simulink model "ControllersComparison"  (R2019b)
settings: Solver=VariableStepAuto  StartTime=0.0  StopTime=tsim  MaxStep=0.01  RelTol=1e-3
values from neighbouring files (symbols this model uses):
  IC = [64.828,     0,  -0.0153, 0,  0,  0,     0, 0,   0,     0,    0, 1119]    [AF_Sim_Init.m]
libraries: simulink_extras x10, simulink x2, aerolibanim x1
settings Model: Creator=Victor  LastModifiedBy=Victor
settings SolverCC: MaxConsecutiveMinStep=50

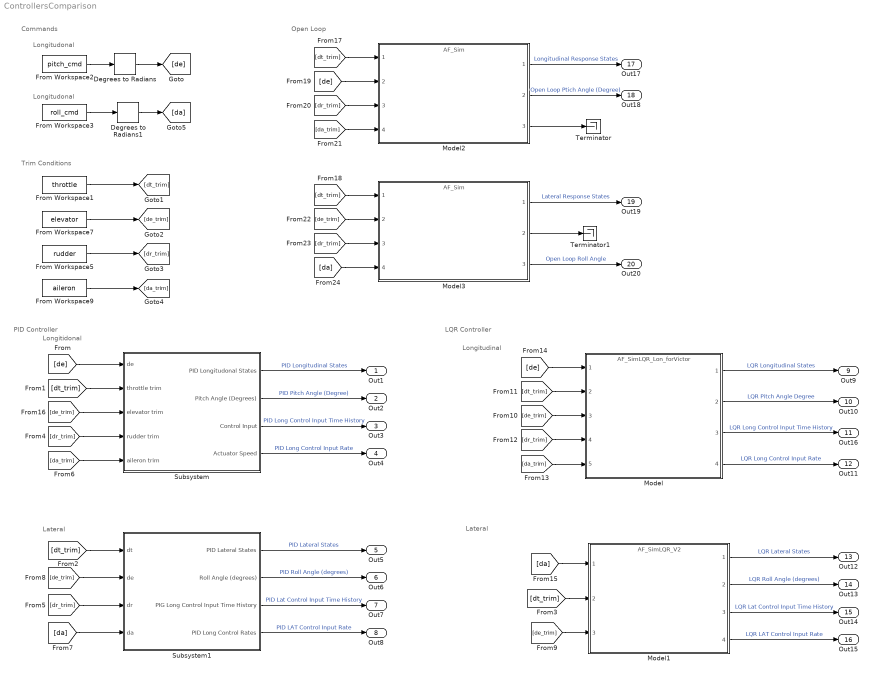
== system ControllersComparison ==
  note: Open Loop
  note: Trim Conditions
  note: Longitudonal
  note: Commands
  note: Longitidonal
  note: PID Controller
  note: Lateral
  note: Longitudinal
  note: LQR Controller
  note: Lateral
  note: Longitudonal
  Degrees to Radians : simulink_extras/Transformations/Degrees to Radians
  Degrees to Radians1 : simulink_extras/Transformations/Degrees to Radians
  From Workspace1 : FromWorkspace  VariableName=throttle  SampleTime=0
  From Workspace2 : FromWorkspace  VariableName=pitch_cmd  SampleTime=0
  From Workspace3 : FromWorkspace  VariableName=roll_cmd  SampleTime=0
  From Workspace5 : FromWorkspace  VariableName=rudder  SampleTime=0
  From Workspace7 : FromWorkspace  VariableName=elevator  SampleTime=0
  From Workspace9 : FromWorkspace  VariableName=aileron  SampleTime=0
  Model : ModelReference  ModelNameDialog=AF_SimLQR_Lon_forVictor.slx  SimulationMode=Normal  ModelReferenceVersion=1.103
  Model1 : ModelReference  ModelNameDialog=AF_SimLQR_V2.slx  SimulationMode=Normal  ModelReferenceVersion=1.56
  Model2 : ModelReference  ModelNameDialog=AF_Sim.slx  SimulationMode=Normal  ModelReferenceVersion=1.35
  Model3 : ModelReference  ModelNameDialog=AF_Sim.slx  SimulationMode=Normal  ModelReferenceVersion=1.35
  Subsystem : Subsystem
  Subsystem1 : Subsystem
  Terminator : Terminator
  Terminator1 : Terminator
  Out1 : Outport
  Out2 : Outport  Port=2
  Out3 : Outport  Port=3
  Out4 : Outport  Port=4
  Out5 : Outport  Port=5
  Out6 : Outport  Port=6
  Out7 : Outport  Port=7
  Out8 : Outport  Port=8
  Out9 : Outport  Port=9
  Out10 : Outport  Port=10
  Out16 : Outport  Port=11
  Out11 : Outport  Port=12
  Out12 : Outport  Port=13
  Out13 : Outport  Port=14
  Out14 : Outport  Port=15
  Out15 : Outport  Port=16
  Out17 : Outport  Port=17
  Out18 : Outport  Port=18
  Out19 : Outport  Port=19
  Out20 : Outport  Port=20
  wires:
  Subsystem/1(PID Longitudonal States) -> Out1/1  "PID Longitudinal States"
  Subsystem/2(Pitch Angle (Degrees)) -> Out2/1  "PID Pitch Angle (Degree)"
  Subsystem/3(Control Input) -> Out3/1  "PID Long Control Input Time History"
  Subsystem/4(Actuator Speed) -> Out4/1  "PID Long Control Input Rate"
  Subsystem1/1(PID Lateral States) -> Out5/1  "PID Lateral States"
  Subsystem1/2(Roll Angle (degrees)) -> Out6/1  "PID Roll Angle (degrees)"
  Subsystem1/3(PIG Long Control Input Time History) -> Out7/1  "PID Lat Control Input Time History"
  Subsystem1/4(PID Long Control Rates) -> Out8/1  "PID LAT Control Input Rate"
  From Workspace2/1 -> Degrees to Radians/1
  Degrees to Radians/1 -> [de]
  [de] -> Subsystem/1(de)
  From Workspace1/1 -> [dt_trim]
  From Workspace7/1 -> [de_trim]
  From Workspace5/1 -> [dr_trim]
  From Workspace9/1 -> [da_trim]
  [dt_trim] -> Subsystem/2(throttle trim)
  [dt_trim] -> Subsystem1/1(dt)
  [dr_trim] -> Subsystem/4(rudder trim)
  [dr_trim] -> Subsystem1/3(dr)
  [da_trim] -> Subsystem/5(aileron trim)
  From Workspace3/1 -> Degrees to Radians1/1
  Degrees to Radians1/1 -> [da]
  [da] -> Subsystem1/4(da)
  [de_trim] -> Subsystem1/2(de)
  [dt_trim] -> Model/2
  [dr_trim] -> Model/4
  [da_trim] -> Model/5
  [de] -> Model/1
  Model/1 -> Out9/1  "LQR Longitudinal States"
  Model/2 -> Out10/1  "LQR Pitch Angle Degree"
  Model/3 -> Out16/1  "LQR Long Control Input Time History"
  Model/4 -> Out11/1  "LQR Long Control Input Rate"
  [de_trim] -> Model/3
  Model1/4 -> Out15/1  "LQR LAT Control Input Rate"
  Model1/3 -> Out14/1  "LQR Lat Control Input Time History"
  Model1/2 -> Out13/1  "LQR Roll Angle (degrees)"
  Model1/1 -> Out12/1  "LQR Lateral States"
  [da] -> Model1/1
  [dt_trim] -> Model1/2
  [de_trim] -> Model1/3
  [de_trim] -> Subsystem/3(elevator trim)
  [dt_trim] -> Model2/1
  [dt_trim] -> Model3/1
  [de] -> Model2/2
  [dr_trim] -> Model2/3
  [da_trim] -> Model2/4
  [de_trim] -> Model3/2
  [dr_trim] -> Model3/3
  [da] -> Model3/4
  Model2/1 -> Out17/1  "Longitudinal Response States"
  Model2/2 -> Out18/1  "Open Loop Ptich Angle (Degree)"
  Model2/3 -> Terminator/1
  Model3/1 -> Out19/1  "Lateral Response States"
  Model3/2 -> Terminator1/1
  Model3/3 -> Out20/1  "Open Loop Roll Angle"

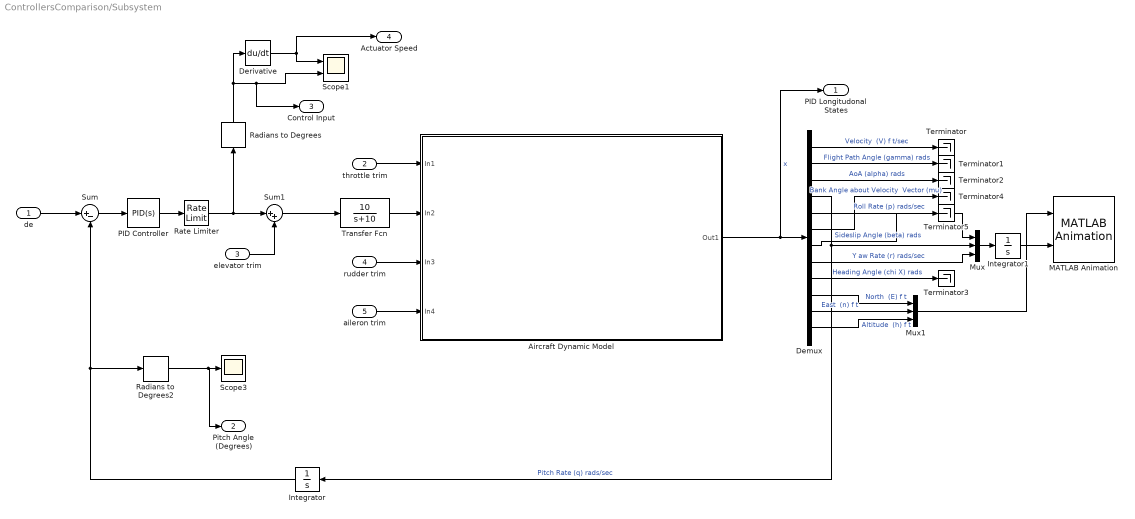
== system ControllersComparison/Subsystem ==
  de : Inport
  throttle trim : Inport  Port=2
  elevator trim : Inport  Port=3
  rudder trim : Inport  Port=4
  aileron trim : Inport  Port=5
  Aircraft Dynamic Model : Subsystem
  Demux : Demux  Outputs=12
  Derivative : Derivative
  Integrator : Integrator
  Integrator1 : Integrator
  MATLAB Animation : aerolibanim/MATLAB Animation  Tag=Matlab Animation 6 DOF  Vehicles=1  Geometries='astredwedge.mat'  BoundingBoxCoordinates=[-50,50,-50,50,-50,50]  CameraOffset=[100,100,100]  CameraViewAngle=4  SampleTime=0.2  FigurePosition=[403,303,275,214]
      settings: SourceProductName=Aerospace Blockset  SourceProductBaseCode=AE
  Mux : Mux  Inputs=3
  Mux1 : Mux  Inputs=3
  PID Controller : simulink/Continuous/PID Controller  Controller=PID  Form=Parallel  TimeDomain=Continuous-time  SampleTime=-1  IntegratorMethod=Forward Euler  FilterMethod=Forward Euler  ControllerParametersSource=internal  P=-1.49308929498648  I=-1.41849985038044  D=-0.103757248214564  UseFilter=on  N=316.418420565516  TunerSelectOption=Transfer Function Based (PID Tuner App)  InitialConditionSource=internal  InitialConditionForIntegrator=0  InitialConditionForFilter=0  DifferentiatorICPrevScaledInput=0  ExternalReset=none  TrackingMode=off  Kt=1  LimitOutput=off  UpperSaturationLimit=12*(pi/180)  LowerSaturationLimit=-12*(pi/180)  LinearizeAsGain=off  AntiWindupMode=back-calculation  Kb=-3  POutMin=[]  POutMax=[]  IOutMin=[]  IOutMax=[]  DOutMin=[]  DOutMax=[]  NOutMin=[]  NOutMax=[]  SumOutMin=[]  SumOutMax=[]  SaturationOutMin=[]  SaturationOutMax=[]  PParamMin=[]  PParamMax=[]  IParamMin=[]  IParamMax=[]  DParamMin=[]  DParamMax=[]  NParamMin=[]  NParamMax=[]  KbParamMin=[]  KbParamMax=[]  KtParamMin=[]  KtParamMax=[]  KbOutMin=[]  KbOutMax=[]  KtOutMin=[]  KtOutMax=[]  IntegratorOutMin=[]  IntegratorOutMax=[]  FilterOutMin=[]  FilterOutMax=[]  SumI1OutMin=[]  SumI1OutMax=[]  SumI2OutMin=[]  SumI2OutMax=[]  SumI3OutMin=[]  SumI3OutMax=[]  SumI4OutMin=[]  SumI4OutMax=[]  SumDOutMin=[]  SumDOutMax=[]  DifferentiatorOutMin=[]  DifferentiatorOutMax=[]  FilterDiffOutCoefMin=[]  FilterDiffOutCoefMax=[]  ReciprocalOutMin=[]  ReciprocalOutMax=[]  SumDenOutMin=[]  SumDenOutMax=[]  SumNumOutMin=[]  SumNumOutMax=[]  DivideOutMin=[]  DivideOutMax=[]  IntegratorContinuousStateAttributes=''  IntegratorStateMustResolveToSignalObject=off  IntegratorRTWStateStorageClass=Auto  FilterContinuousStateAttributes=''  FilterStateMustResolveToSignalObject=off  FilterRTWStateStorageClass=Auto  ParallelPVariant=InternalParameters  IdealPVariant=Disabled  IVariant=InternalParameters  DVariant=InternalParameters  IntegratorVariant=Continuous  SatVariant=Disabled  AWVariant=Passthrough  PCopyVariant=Disabled  TRVariant=Disabled  FdbkBlocksVariant=Forward  IdealPFdbkVariant=Disabled  SatFdbkVariant=Disabled  DerivativeFilterVariant=ContFilter  NVariant=InternalParameters  NCopyVariant=Disabled  FilterICVariant=InternalICsFilter  IntegratorICVariant=InternalICs  ExternalResetVariant=Disabled  TRSumVariant=Passthrough  SumFdbkVariant=Disabled  SumVariant=Sum_PID
  Radians to Degrees : simulink_extras/Transformations/Radians to Degrees
  Radians to Degrees2 : simulink_extras/Transformations/Radians to Degrees
  Rate Limiter : RateLimiter  RisingSlewLimit=10  FallingSlewLimit=-10  SampleTimeMode=inherited
  Scope1 : Scope  NumInputPorts=2
  Scope3 : Scope
  Sum : Sum  Inputs=|+-
  Sum1 : Sum  Inputs=|++
  Terminator{,1..5} (6 alike) : Terminator
  Transfer Fcn : TransferFcn  Numerator=[10]  Denominator=[1 10]
  PID Longitudonal States : Outport
  Pitch Angle (Degrees) : Outport  Port=2
  Control Input : Outport  Port=3
  Actuator Speed : Outport  Port=4
  wires:
  Aircraft Dynamic Model/1(Out1) -> PID Longitudonal States/1, Demux/1  "x"
  Demux/4 -> Integrator/1, Mux/2  "Pitch Rate (q) rads/sec"
  Sum/1 -> PID Controller/1
  Transfer Fcn/1 -> Aircraft Dynamic Model/2(In2)
  Derivative/1 -> Scope1/1, Actuator Speed/1
  Radians to Degrees/1 -> Derivative/1, Control Input/1, Scope1/2
  rudder trim/1 -> Aircraft Dynamic Model/3(In3)
  aileron trim/1 -> Aircraft Dynamic Model/4(In4)
  throttle trim/1 -> Aircraft Dynamic Model/1(In1)
  de/1 -> Sum/1
  Integrator/1 -> Sum/2, Radians to Degrees2/1
  Radians to Degrees2/1 -> Pitch Angle (Degrees)/1, Scope3/1
  Demux/5 -> Mux/1  "Roll Rate (p) rads/sec"
  Demux/8 -> Mux/3  "Y aw Rate (r) rads/sec"
  Mux/1 -> Integrator1/1
  Integrator1/1 -> MATLAB Animation/2
  Demux/10 -> Mux1/1  "North  (E) f t"
  Demux/11 -> Mux1/2  "East  (n) f t"
  Demux/12 -> Mux1/3  "Altitude  (h) f t"
  Mux1/1 -> MATLAB Animation/1
  Sum1/1 -> Transfer Fcn/1
  Demux/1 -> Terminator/1  "Velocity  (V) f t/sec"
  Demux/2 -> Terminator1/1  "Flight Path Angle (gamma) rads"
  Demux/3 -> Terminator2/1  "AoA (alpha) rads"
  Demux/9 -> Terminator3/1  "Heading Angle (chi X) rads"
  Demux/6 -> Terminator4/1  "Bank Angle about Velocity  Vector (mu)"
  Demux/7 -> Terminator5/1  "Sideslip Angle (beta) rads"
  elevator trim/1 -> Sum1/2
  Rate Limiter/1 -> Radians to Degrees/1, Sum1/1
  PID Controller/1 -> Rate Limiter/1

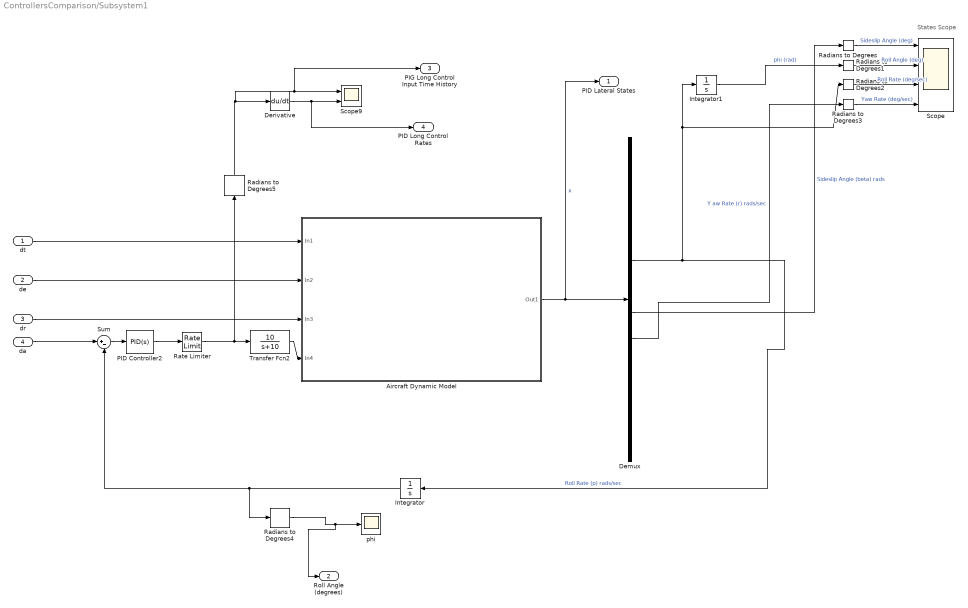
== system ControllersComparison/Subsystem1 ==
  note: States Scope
  dt : Inport
  de : Inport  Port=2
  dr : Inport  Port=3
  da : Inport  Port=4
  Aircraft Dynamic Model : Subsystem
  Demux : Demux  Outputs=12
  Derivative : Derivative
  Integrator : Integrator
  Integrator1 : Integrator
  PID Controller2 : simulink/Continuous/PID Controller  Controller=PID  Form=Parallel  TimeDomain=Continuous-time  SampleTime=-1  IntegratorMethod=Forward Euler  FilterMethod=Forward Euler  ControllerParametersSource=internal  P=1.61606482849741  I=1.22173294294368  D=0.356576763881949  UseFilter=on  N=1149.82034893271  TunerSelectOption=Transfer Function Based (PID Tuner App)  InitialConditionSource=internal  InitialConditionForIntegrator=0  InitialConditionForFilter=0  DifferentiatorICPrevScaledInput=0  ExternalReset=none  TrackingMode=off  Kt=1  LimitOutput=off  UpperSaturationLimit=inf  LowerSaturationLimit=-inf  LinearizeAsGain=on  AntiWindupMode=none  Kb=1  POutMin=[]  POutMax=[]  IOutMin=[]  IOutMax=[]  DOutMin=[]  DOutMax=[]  NOutMin=[]  NOutMax=[]  SumOutMin=[]  SumOutMax=[]  SaturationOutMin=[]  SaturationOutMax=[]  PParamMin=[]  PParamMax=[]  IParamMin=[]  IParamMax=[]  DParamMin=[]  DParamMax=[]  NParamMin=[]  NParamMax=[]  KbParamMin=[]  KbParamMax=[]  KtParamMin=[]  KtParamMax=[]  KbOutMin=[]  KbOutMax=[]  KtOutMin=[]  KtOutMax=[]  IntegratorOutMin=[]  IntegratorOutMax=[]  FilterOutMin=[]  FilterOutMax=[]  SumI1OutMin=[]  SumI1OutMax=[]  SumI2OutMin=[]  SumI2OutMax=[]  SumI3OutMin=[]  SumI3OutMax=[]  SumI4OutMin=[]  SumI4OutMax=[]  SumDOutMin=[]  SumDOutMax=[]  DifferentiatorOutMin=[]  DifferentiatorOutMax=[]  FilterDiffOutCoefMin=[]  FilterDiffOutCoefMax=[]  ReciprocalOutMin=[]  ReciprocalOutMax=[]  SumDenOutMin=[]  SumDenOutMax=[]  SumNumOutMin=[]  SumNumOutMax=[]  DivideOutMin=[]  DivideOutMax=[]  IntegratorContinuousStateAttributes=''  IntegratorStateMustResolveToSignalObject=off  IntegratorRTWStateStorageClass=Auto  FilterContinuousStateAttributes=''  FilterStateMustResolveToSignalObject=off  FilterRTWStateStorageClass=Auto  ParallelPVariant=InternalParameters  IdealPVariant=Disabled  IVariant=InternalParameters  DVariant=InternalParameters  IntegratorVariant=Continuous  SatVariant=Disabled  AWVariant=Passthrough  PCopyVariant=Disabled  TRVariant=Disabled  FdbkBlocksVariant=Forward  IdealPFdbkVariant=Disabled  SatFdbkVariant=Disabled  DerivativeFilterVariant=ContFilter  NVariant=InternalParameters  NCopyVariant=Disabled  FilterICVariant=InternalICsFilter  IntegratorICVariant=InternalICs  ExternalResetVariant=Disabled  TRSumVariant=Passthrough  SumFdbkVariant=Disabled  SumVariant=Sum_PID
  Radians to Degrees{,1..5} (6 alike) : simulink_extras/Transformations/Radians to Degrees
  Rate Limiter : RateLimiter  RisingSlewLimit=10  FallingSlewLimit=-10  SampleTimeMode=inherited
  Scope : Scope  NumInputPorts=4
  Scope9 : Scope  NumInputPorts=2
  Sum : Sum  Inputs=|+-
  Transfer Fcn2 : TransferFcn  Numerator=[10]  Denominator=[1 10]
  phi : Scope
  PID Lateral States : Outport
  Roll Angle (degrees) : Outport  Port=2
  PIG Long Control Input Time History : Outport  Port=3
  PID Long Control Rates : Outport  Port=4
  wires:
  Demux/8 -> Radians to Degrees3/1  "Y aw Rate (r) rads/sec"
  Aircraft Dynamic Model/1(Out1) -> PID Lateral States/1, Demux/1  "x"
  Rate Limiter/1 -> Transfer Fcn2/1, Radians to Degrees5/1
  Derivative/1 -> PID Long Control Rates/1, Scope9/2
  Demux/5 -> Radians to Degrees2/1, Integrator1/1, Integrator/1  "Roll Rate (p) rads/sec"
  dt/1 -> Aircraft Dynamic Model/1(In1)
  Demux/7 -> Radians to Degrees/1  "Sideslip Angle (beta) rads"
  Radians to Degrees4/1 -> Roll Angle (degrees)/1, phi/1
  Integrator1/1 -> Radians to Degrees1/1  "phi (rad)"
  dr/1 -> Aircraft Dynamic Model/3(In3)
  Radians to Degrees3/1 -> Scope/4  "Yaw Rate (deg/sec)"
  Radians to Degrees1/1 -> Scope/2  "Roll Angle (deg)"
  Radians to Degrees/1 -> Scope/1  "Sideslip Angle (deg)"
  Transfer Fcn2/1 -> Aircraft Dynamic Model/4(In4)
  de/1 -> Aircraft Dynamic Model/2(In2)
  Radians to Degrees2/1 -> Scope/3  "Roll Rate (deg/sec)"
  Sum/1 -> PID Controller2/1
  PID Controller2/1 -> Rate Limiter/1
  Integrator/1 -> Radians to Degrees4/1, Sum/2
  da/1 -> Sum/1
  Radians to Degrees5/1 -> Derivative/1, PIG Long Control Input Time History/1, Scope9/1

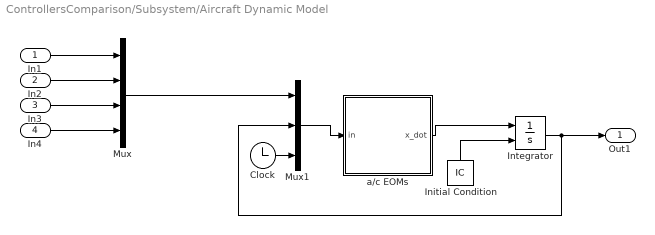
== system ControllersComparison/Subsystem/Aircraft Dynamic Model ==
  In1 : Inport
  In2 : Inport  Port=2
  In3 : Inport  Port=3
  In4 : Inport  Port=4
  Clock : Clock
      settings: Decimation=100
  Initial Condition : Constant  Value=IC
  Integrator : Integrator  InitialConditionSource=external
  Mux : Mux
  Mux1 : Mux  Inputs=3
  a/c EOMs : MATLAB Function  TreatAsAtomicUnit=on
  Out1 : Outport  VectorParamsAs1DForOutWhenUnconnected=off
  wires:
  Initial Condition/1 -> Integrator/2
  Clock/1 -> Mux1/3
  Integrator/1 -> Mux1/2, Out1/1
  Mux1/1 -> a/c EOMs/1(in)
  a/c EOMs/1(x_dot) -> Integrator/1
  Mux/1 -> Mux1/1
  In1/1 -> Mux/1
  In2/1 -> Mux/2
  In3/1 -> Mux/3
  In4/1 -> Mux/4

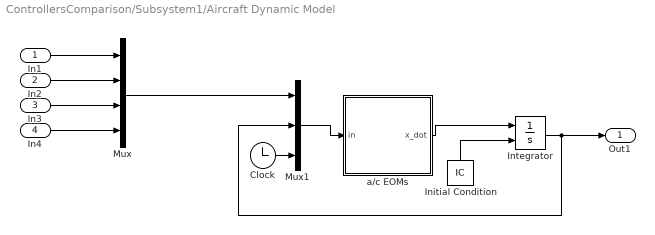
== system ControllersComparison/Subsystem1/Aircraft Dynamic Model ==
  In1 : Inport
  In2 : Inport  Port=2
  In3 : Inport  Port=3
  In4 : Inport  Port=4
  Clock : Clock
      settings: Decimation=100
  Initial Condition : Constant  Value=IC
  Integrator : Integrator  InitialConditionSource=external
  Mux : Mux
  Mux1 : Mux  Inputs=3
  a/c EOMs : MATLAB Function  TreatAsAtomicUnit=on
  Out1 : Outport  VectorParamsAs1DForOutWhenUnconnected=off
  wires:
  a/c EOMs/1(x_dot) -> Integrator/1
  In3/1 -> Mux/3
  Clock/1 -> Mux1/3
  Integrator/1 -> Mux1/2, Out1/1
  Initial Condition/1 -> Integrator/2
  Mux/1 -> Mux1/1
  Mux1/1 -> a/c EOMs/1(in)
  In4/1 -> Mux/4
  In2/1 -> Mux/2
  In1/1 -> Mux/1

== matlab function ControllersComparison/Subsystem1/Aircraft Dynamic Model/a//c EOMs ==
  data: in input; x_dot output
function x_dot  = fcn(in)

%global manuever alpha_dot;
x_dot = zeros(12,1);

alpha_dot = 0;

%temporary input vector
%u0 = [1.29, -0.1174, 0,  0, 64.828,     0,  -0.0153, 0,  0,  0,     0, 0,   0,     0,    0, 1119, 100];
    % [T,     de,    dr, da, V,      gamma,  AoA,     q,  p, mu,  beta, r, chi, north, east,    h, clock-input]
  
%in = u0;

% PARSING INPUTS
%=============================================================
T   = in(1); %Thrust
de  = in(2); %Elevator deflection (down is +) {deg}
drt = in(3); %Rudder deflection {deg}
da  = in(4); %Aileron deflection {deg}

V       = in(5);  %Velocity {ft/s}
gamma   = in(6);  %Flight path angle {rad}
alpha   = in(7);  %Angle of attack {rad}
q       = in(8);  %Pitch Rate {rad/s}
p       = in(9);  %Roll Rate {rad/s}
mu      = in(10); %Bank Angle (About Velocity Vector) {rad}
beta    = in(11); %Sideslip Angle {rad}
r       = in(12); %Yaw Rate {rad/s}
chi     = in(13); %Heading angle {rads}
north   = in(14); %North Position {ft}
east    = in(15); %East Position {ft}
h       = in(16); %Altitude {ft}
tm = in(17); % time {s}

% ATMOSPHERIC PROPERTIES
%=============================================================
rho = 0.0023081;    %Air Density (slugs per ft^3) -> do we want to make this a function of height?
g = 32.17;          %ft/s^2


% AIRCRAFT PROPERTIES
%==============================================================


m = 0.487669;       %Slugs - empty mass w/o fuel
Iyy = 1.5523;       %Inertia found with empty mass
Ixx = 1.948;        %Inertia
Izz = 1.9166;       %Inertia
Ixz = 0;            %Assumed zero due to symmetric aircraft

S = 10.56;          %Wing area - square feet
b = 9.16;           % Wing span - feet

CLow = 0.421;       %Wing coefficient of lift at 0deg AoA
CLaw = 4.59;        %Wing coefficient of lift per AoA
CDminw = 0.011;     %wing minimum coefficient of drag
ARw = (b^2)/S;      %Wing aspect ratio
e = 0.75;           %Span efficiency - ESTIMATION
Kw = 1/(pi*ARw*e);  %
Cmw = -0.005;       %Wing moment coefficient
cgw = -(5/12);      %Distance aero center is back from cg - 5 inches
c = (16/12);        %Root chord of wing (16") - feet
lambda = 0.72955;   %Taper ratio from S = (Cr*(1+lambda)*b)/2
CLat = 0.76;        %Vert tail coefficient of lift per AoA
CDmint = 0.002;     %vert tail minimum coeffcient of drag
Kt = 0.446;         %TO DO - MORE CALC?
it = deg2rad(2);    %Tail incidence 2 degrees to radians
Te = 0.422;         %Tail control surface effectiveness (??)
nt = 1;             %??
St = S;             %Horizontal tail area square feet = ref area (??)
cgt = 3.5;          %Distance tail aero center back from a/c cg

CLavt = 0.0969;     %Vertical tail coefficient of lift per AoA(??)
CDminvt = 0.001;    %vert tail min coefficient of drag (??)
Svt = S;            %Ref area of vertical tail = ref area (??)
Tr = 0.434;         %Name??
nvt = nt;           %same as hori tail (??)
cgvt = cgt;         %same as hori tail (??)

Cmaf = 0.114;       %fuselage moment coefficient
CDf = 0.005;        %Fuselage coefficient of drag

Cnda = -0.0128;     %per rad (??)
Clda = 0.244;       %per rad (??)

%Eqns 17-25
CLw=CLow+CLaw*alpha;
CDw=CDminw+Kw*CLw^2;
E=2*(CLow+CLaw*(alpha-alpha_dot*(cgt+cgw)/V))/(pi*ARw);
alphat=alpha+it+Te*de+q*cgt/V-E;
CLt=CLat*alphat;
CDt=CDmint+Kt*CLt^2;
Cmf=Cmaf*alpha;
CDvt=CDminvt;
Clp=-1/12*CLaw*(1+3*lambda)/(1+lambda);

Clb=-.1;
Clr=.01;

%Eqns 26 - 33
qb=.5*rho*V^2;
Lw=qb*S*CLw;
Dw=qb*S*CDw;
Mw=qb*S*c*Cmw;
Lt=nt*qb*St*CLt;
Dt=nt*qb*St*CDt;
Df=qb*S*CDf;
Mf=qb*S*c*Cmf;
Dvt=nt*qb*Svt*CDvt;

% Calculate Forces and Moments
% Lift
L=Lw+Lt*cos(E-q*cgt/V)-(Dt+Dvt)*sin(E-q*cgt/V);
% Drag
D=Dw+(Dt+Dvt)*cos(E-q*cgt/V)+Lt*sin(E-q*cgt/V)+Df;
% Side Force
Y=nvt*qb*Svt*CLavt*(-beta+Tr*drt+r*cgvt/V);
% Pitch Moment
Mc=Lw*cgw*cos(alpha)+Dw*cgw*sin(alpha)+Mw-Lt*cgt*cos(alpha-E+q*cgt/V)-(Dt+Dvt)*cgt*sin(alpha-E+q*cgt/V)+Mf;
% Yaw Moment
Nc=-qb*nvt*Svt*CLavt*(-beta+Tr*drt+r*cgvt/V)*cgvt+(-qb*S*b*Cnda*da);
% Roll Moment
Lc=qb*S*b^2/(2*V)*(Clp*p+2*V/b*Clb*beta+Clr*drt+Clda*da*2*V/b);

% -=-=-=-=-=- NONLINEAR 6-DOF EQUATION OF MOTION (EOMs) -=-=-=-=-=-=-=-=-
%
% These are the state derivative equations; the comment names the state,
% but the equation is for its derivative (rate)
%
% The equations are arranged by aircraft mode
%
% NOTE: These assume that Ixz=0, if not, then eq's need to be modified
% Longitudinal (phugoid and short period): V, gamma, q, alpha
% Phugoid: V, gamma
 % Velocity
 V_dot=1/m*(-D*cos(beta)+Y*sin(beta)+T*cos(beta)*cos(alpha))-...
 g*sin(gamma);
 % Flight Path Angle
 gamma_dot=1/(m*V)*(-D*sin(beta)*sin(mu)-Y*sin(mu)*cos(beta)...
 +L*cos(mu)+T*(cos(mu)*sin(alpha)+sin(mu)*sin(beta)*cos(alpha)))...
 -g/V*cos(gamma);
% Short Period: alpha, q
 % Angle of Attach
 alpha_dot=q-tan(beta)*(p*cos(alpha)+r*sin(alpha))-1/(m*V*cos(beta))...
 *(L+T*sin(alpha))+g*cos(gamma)*cos(mu)/(V*cos(beta));
 % Pitch Rate
 q_dot=Mc/Iyy+1/Iyy*(Izz*p*r-Ixx*r*p);
% Lateral (roll) - Directional (yaw): p, mu, beta, r
% Roll: p, mu
 % Roll Rate
 p_dot=Lc/Ixx+1/Ixx*(Iyy*r*q-Izz*q*r);

 % Bank Angle (about velocity vector)
 mu_dot=1/cos(beta)*(p*cos(alpha)+r*sin(alpha))+1/(m*V)*(D*sin(beta)...
 *cos(mu)*tan(gamma)+Y*tan(gamma)*cos(mu)*cos(beta)+L*(tan(beta)+...
 tan(gamma)*sin(mu))+T*(sin(alpha)*tan(gamma)*sin(mu)+sin(alpha)*...
 tan(beta)-cos(alpha)*tan(gamma)*cos(mu)*sin(beta)))-...
 g/V*cos(gamma)*cos(mu)*tan(beta);

% Dutch Roll: beta, r
 % Side Slip Angle
 beta_dot=-r*cos(alpha)+p*sin(alpha)+1/(m*V)*(D*sin(beta)+Y*cos...
 (beta)-T*sin(beta)*cos(alpha))+g/V*cos(gamma)*sin(mu);

 % Yaw Rate

 r_dot=Nc/Izz+1/Izz*(Ixx*p*q-Iyy*p*q);

% Heading Angle (from North)
 chi_dot=1/(m*V*cos(gamma))*(D*sin(beta)*cos(mu)+Y*cos(mu)*cos(beta)...
 +L*sin(mu)+T*(sin(mu)*sin(alpha)-cos(mu)*sin(beta)*cos(alpha)));

% Kinematic Equations
 % North Position
 n_dot=V*cos(gamma)*cos(chi);

 % East Position
 e_dot=V*cos(gamma)*sin(chi);

 % Altitude
 h_dot=V*sin(gamma);

% Pack derivatives into output vector x_dot
 x_dot(1) = V_dot;
 x_dot(2) = gamma_dot;
 x_dot(3) = alpha_dot;
 x_dot(4) = q_dot;
 x_dot(5) = p_dot;
 x_dot(6) = mu_dot;
 x_dot(7) = beta_dot;
 x_dot(8) = r_dot;
 x_dot(9) = chi_dot;
 x_dot(10) = n_dot;
 x_dot(11) = e_dot;
 x_dot(12) = h_dot;
 
end

== matlab function ControllersComparison/Subsystem/Aircraft Dynamic Model/a//c EOMs ==
  data: in input; x_dot output
function x_dot  = fcn(in)

%global manuever alpha_dot;
x_dot = zeros(12,1);

alpha_dot = 0;

%temporary input vector
%u0 = [1.29, -0.1174, 0,  0, 64.828,     0,  -0.0153, 0,  0,  0,     0, 0,   0,     0,    0, 1119, 100];
    % [T,     de,    dr, da, V,      gamma,  AoA,     q,  p, mu,  beta, r, chi, north, east,    h, clock-input]
  
%in = u0;

% PARSING INPUTS
%=============================================================
T   = in(1); %Thrust
de  = in(2); %Elevator deflection (down is +) {deg}
drt = in(3); %Rudder deflection {deg}
da  = in(4); %Aileron deflection {deg}

V       = in(5);  %Velocity {ft/s}
gamma   = in(6);  %Flight path angle {rad}
alpha   = in(7);  %Angle of attack {rad}
q       = in(8);  %Pitch Rate {rad/s}
p       = in(9);  %Roll Rate {rad/s}
mu      = in(10); %Bank Angle (About Velocity Vector) {rad}
beta    = in(11); %Sideslip Angle {rad}
r       = in(12); %Yaw Rate {rad/s}
chi     = in(13); %Heading angle {rads}
north   = in(14); %North Position {ft}
east    = in(15); %East Position {ft}
h       = in(16); %Altitude {ft}
tm = in(17); % time {s}

% ATMOSPHERIC PROPERTIES
%=============================================================
rho = 0.0023081;    %Air Density (slugs per ft^3) -> do we want to make this a function of height?
g = 32.17;          %ft/s^2


% AIRCRAFT PROPERTIES
%==============================================================


m = 0.487669;       %Slugs - empty mass w/o fuel
Iyy = 1.5523;       %Inertia found with empty mass
Ixx = 1.948;        %Inertia
Izz = 1.9166;       %Inertia
Ixz = 0;            %Assumed zero due to symmetric aircraft

S = 10.56;          %Wing area - square feet
b = 9.16;           % Wing span - feet

CLow = 0.421;       %Wing coefficient of lift at 0deg AoA
CLaw = 4.59;        %Wing coefficient of lift per AoA
CDminw = 0.011;     %wing minimum coefficient of drag
ARw = (b^2)/S;      %Wing aspect ratio
e = 0.75;           %Span efficiency - ESTIMATION
Kw = 1/(pi*ARw*e);  %
Cmw = -0.005;       %Wing moment coefficient
cgw = -(5/12);      %Distance aero center is back from cg - 5 inches
c = (16/12);        %Root chord of wing (16") - feet
lambda = 0.72955;   %Taper ratio from S = (Cr*(1+lambda)*b)/2
CLat = 0.76;        %Vert tail coefficient of lift per AoA
CDmint = 0.002;     %vert tail minimum coeffcient of drag
Kt = 0.446;         %TO DO - MORE CALC?
it = deg2rad(2);    %Tail incidence 2 degrees to radians
Te = 0.422;         %Tail control surface effectiveness (??)
nt = 1;             %??
St = S;             %Horizontal tail area square feet = ref area (??)
cgt = 3.5;          %Distance tail aero center back from a/c cg

CLavt = 0.0969;     %Vertical tail coefficient of lift per AoA(??)
CDminvt = 0.001;    %vert tail min coefficient of drag (??)
Svt = S;            %Ref area of vertical tail = ref area (??)
Tr = 0.434;         %Name??
nvt = nt;           %same as hori tail (??)
cgvt = cgt;         %same as hori tail (??)

Cmaf = 0.114;       %fuselage moment coefficient
CDf = 0.005;        %Fuselage coefficient of drag

Cnda = -0.0128;     %per rad (??)
Clda = 0.244;       %per rad (??)

%Eqns 17-25
CLw=CLow+CLaw*alpha;
CDw=CDminw+Kw*CLw^2;
E=2*(CLow+CLaw*(alpha-alpha_dot*(cgt+cgw)/V))/(pi*ARw);
alphat=alpha+it+Te*de+q*cgt/V-E;
CLt=CLat*alphat;
CDt=CDmint+Kt*CLt^2;
Cmf=Cmaf*alpha;
CDvt=CDminvt;
Clp=-1/12*CLaw*(1+3*lambda)/(1+lambda);

Clb=-.1;
Clr=.01;

%Eqns 26 - 33
qb=.5*rho*V^2;
Lw=qb*S*CLw;
Dw=qb*S*CDw;
Mw=qb*S*c*Cmw;
Lt=nt*qb*St*CLt;
Dt=nt*qb*St*CDt;
Df=qb*S*CDf;
Mf=qb*S*c*Cmf;
Dvt=nt*qb*Svt*CDvt;

% Calculate Forces and Moments
% Lift
L=Lw+Lt*cos(E-q*cgt/V)-(Dt+Dvt)*sin(E-q*cgt/V);
% Drag
D=Dw+(Dt+Dvt)*cos(E-q*cgt/V)+Lt*sin(E-q*cgt/V)+Df;
% Side Force
Y=nvt*qb*Svt*CLavt*(-beta+Tr*drt+r*cgvt/V);
% Pitch Moment
Mc=Lw*cgw*cos(alpha)+Dw*cgw*sin(alpha)+Mw-Lt*cgt*cos(alpha-E+q*cgt/V)-(Dt+Dvt)*cgt*sin(alpha-E+q*cgt/V)+Mf;
% Yaw Moment
Nc=-qb*nvt*Svt*CLavt*(-beta+Tr*drt+r*cgvt/V)*cgvt+(-qb*S*b*Cnda*da);
% Roll Moment
Lc=qb*S*b^2/(2*V)*(Clp*p+2*V/b*Clb*beta+Clr*drt+Clda*da*2*V/b);

% -=-=-=-=-=- NONLINEAR 6-DOF EQUATION OF MOTION (EOMs) -=-=-=-=-=-=-=-=-
%
% These are the state derivative equations; the comment names the state,
% but the equation is for its derivative (rate)
%
% The equations are arranged by aircraft mode
%
% NOTE: These assume that Ixz=0, if not, then eq's need to be modified
% Longitudinal (phugoid and short period): V, gamma, q, alpha
% Phugoid: V, gamma
 % Velocity
 V_dot=1/m*(-D*cos(beta)+Y*sin(beta)+T*cos(beta)*cos(alpha))-...
 g*sin(gamma);
 % Flight Path Angle
 gamma_dot=1/(m*V)*(-D*sin(beta)*sin(mu)-Y*sin(mu)*cos(beta)...
 +L*cos(mu)+T*(cos(mu)*sin(alpha)+sin(mu)*sin(beta)*cos(alpha)))...
 -g/V*cos(gamma);
% Short Period: alpha, q
 % Angle of Attach
 alpha_dot=q-tan(beta)*(p*cos(alpha)+r*sin(alpha))-1/(m*V*cos(beta))...
 *(L+T*sin(alpha))+g*cos(gamma)*cos(mu)/(V*cos(beta));
 % Pitch Rate
 q_dot=Mc/Iyy+1/Iyy*(Izz*p*r-Ixx*r*p);
% Lateral (roll) - Directional (yaw): p, mu, beta, r
% Roll: p, mu
 % Roll Rate
 p_dot=Lc/Ixx+1/Ixx*(Iyy*r*q-Izz*q*r);

 % Bank Angle (about velocity vector)
 mu_dot=1/cos(beta)*(p*cos(alpha)+r*sin(alpha))+1/(m*V)*(D*sin(beta)...
 *cos(mu)*tan(gamma)+Y*tan(gamma)*cos(mu)*cos(beta)+L*(tan(beta)+...
 tan(gamma)*sin(mu))+T*(sin(alpha)*tan(gamma)*sin(mu)+sin(alpha)*...
 tan(beta)-cos(alpha)*tan(gamma)*cos(mu)*sin(beta)))-...
 g/V*cos(gamma)*cos(mu)*tan(beta);

% Dutch Roll: beta, r
 % Side Slip Angle
 beta_dot=-r*cos(alpha)+p*sin(alpha)+1/(m*V)*(D*sin(beta)+Y*cos...
 (beta)-T*sin(beta)*cos(alpha))+g/V*cos(gamma)*sin(mu);

 % Yaw Rate

 r_dot=Nc/Izz+1/Izz*(Ixx*p*q-Iyy*p*q);

% Heading Angle (from North)
 chi_dot=1/(m*V*cos(gamma))*(D*sin(beta)*cos(mu)+Y*cos(mu)*cos(beta)...
 +L*sin(mu)+T*(sin(mu)*sin(alpha)-cos(mu)*sin(beta)*cos(alpha)));

% Kinematic Equations
 % North Position
 n_dot=V*cos(gamma)*cos(chi);

 % East Position
 e_dot=V*cos(gamma)*sin(chi);

 % Altitude
 h_dot=V*sin(gamma);

% Pack derivatives into output vector x_dot
 x_dot(1) = V_dot;
 x_dot(2) = gamma_dot;
 x_dot(3) = alpha_dot;
 x_dot(4) = q_dot;
 x_dot(5) = p_dot;
 x_dot(6) = mu_dot;
 x_dot(7) = beta_dot;
 x_dot(8) = r_dot;
 x_dot(9) = chi_dot;
 x_dot(10) = n_dot;
 x_dot(11) = e_dot;
 x_dot(12) = h_dot;
 
end
